simulink model "Lab1_2_encoder"  (Simulink 7.3)
settings: Solver=ode3  StartTime=0.0  StopTime=10.0  FixedStep=0.001  RelTol=1e-3
undefined symbols (not defined in the file or in its folder): MultiQ, PCI, Quanser
libraries: rtwinlib x3
settings Model: Creator=Mehatronicki Sustavi  LastModifiedBy=Mehatronicki Sustavi  SimulationMode=external  ExtModeTrigDuration=1000000
settings HardwareCC: ProdIntDivRoundTo=Zero  ProdEndianess=LittleEndian  ProdHWDeviceType=Generic->32-bit x86 compatible
settings RTWCC: SystemTargetFile=rtwin.tlc  TemplateMakefile=rtwin.tmf  Description=Real-Time Windows Target  ProcessScript=rtwin_make_rtw_hook  RTWCompilerOptimization=On
settings CodeAppCC: MaxIdLength=95
settings RTWinTargetCC: TargetLibSuffix=_rtwin.lib  TargetPreCompLibLocation=C:\Program Files\MATLAB\R2009a\toolbox\rtw\targets\rtwin\lib  TargetFunctionLibrary=ANSI_C  PortableWordSizes=off

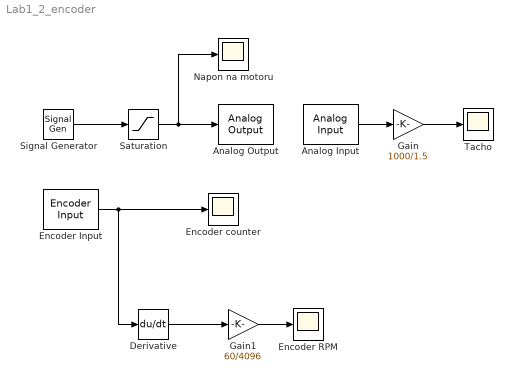
== system Lab1_2_encoder ==
  Analog Input : rtwinlib/Analog Input  SampleTime=0.001  DrvName=Quanser/MultiQ-PCI  DrvAddress=4294967295  DrvOptions=zeros(1,0)  Channels=2  RangeMode=1  VoltRange=1  DataType=1
      settings: AttributesFormatString=Quanser\nMultiQ-PCI [auto]
  Analog Output : rtwinlib/Analog Output  SampleTime=0.001  DrvName=Quanser/MultiQ-PCI  DrvAddress=4294967295  DrvOptions=zeros(1,0)  Channels=1  RangeMode=1  VoltRange=1  InitialValue=0  FinalValue=0
      settings: AttributesFormatString=Quanser\nMultiQ-PCI [auto]
  Derivative : Derivative  LinearizePole=0.0001
  Encoder Input : rtwinlib/Encoder Input  SampleTime=0.001  DrvName=Quanser/MultiQ-PCI  DrvAddress=4294967295  DrvOptions=zeros(1,0)  Channels=1  QuadMode=3  IndexPulse=2  InputFilter=Inf  DataType=1
      settings: AttributesFormatString=Quanser\nMultiQ-PCI [auto]
  Encoder RPM : Scope
      settings: YMin=-5000  YMax=5000  SaveName=EncoderRPM  DataFormat=Array
  Encoder counter : Scope
      settings: YMin=0  YMax=12000  SaveName=EncoderCnt  DataFormat=Array
  Gain : Gain  Gain=1000/1.5  ParameterDataType=fixdt(1, 16)  ParameterScaling=2^0  OutDataType=fixdt(1, 16)  OutScaling=2^0
  Gain1 : Gain  Gain=60/4096  ParameterDataType=fixdt(1, 16)  ParameterScaling=2^0  OutDataType=fixdt(1, 16)  OutScaling=2^0
  Napon na motoru : Scope
      settings: SaveName=NaponMotor  DataFormat=Array
  Saturation : Saturate  UpperLimit=6  LowerLimit=-6  OutDataType=fixdt(1, 16)  OutScaling=2^0
  Signal Generator : SignalGenerator  WaveForm=square  Amplitude=3  Frequency=0.1
  Tacho : Scope
      settings: YMin=-3500  YMax=3500  SaveName=Tacho  DataFormat=Array
  wires:
  Signal Generator/1 -> Saturation/1
  Saturation/1 -> Analog Output/1, Napon na motoru/1
  Analog Input/1 -> Gain/1
  Gain/1 -> Tacho/1
  Encoder Input/1 -> Derivative/1, Encoder counter/1
  Derivative/1 -> Gain1/1
  Gain1/1 -> Encoder RPM/1
